simulink model "CHinf"  (R2020b)
settings: Solver=ode45  StartTime=0.0  StopTime=10  FixedStep=0.01  MaxStep=0.01  RelTol=1e-3  EnableMultiTasking=on
undefined symbols (not defined in the file): B, J, K1, Ke, Kt, Ra
settings Model: Creator=Harryth  LastModifiedBy=andre
settings DataIOCC: LimitDataPoints=on  SaveFormat=Array  SignalLoggingSaveFormat=ModelDataLogs  ReturnWorkspaceOutputs=off
settings OptimizationCC: ExpressionDepthLimit=2147483647  LifeSpan=inf
settings DebuggingCC: UnderspecifiedInitializationDetection=Classic  MergeDetectMultiDrivingBlocksExec=none  SolverPrmCheckMsg=warning  FcnCallInpInsideContextMsg=warning  StateNameClashWarn=warning  SFUnexpectedBacktrackingDiag=warning  SFNoUnconditionalDefaultTransitionDiag=warning  SFExecutionAtInitializationDiag=none  ArithmeticOperatorsInVariantConditions=warning
settings HardwareCC: ProdBitPerPointer=32  ProdBitPerSizeT=32  ProdBitPerPtrDiffT=32  ProdLargestAtomicFloat=None  ProdIntDivRoundTo=Undefined  ProdEndianess=Unspecified  ProdWordSize=32  ProdHWDeviceType=32-bit Generic
settings ModelReferenceCC: PropagateSignalLabelsOutOfModel=off
settings SFSimCC: SimUseLocalCustomCode=off  CustomCodeUndefinedFunction=UseInterfaceOnly
settings RTWCC: RTWUseLocalCustomCode=off
settings CodeAppCC: StateflowObjectComments=on
settings GRTTargetCC: TargetLangStandard=C89/C90 (ANSI)  CombineOutputUpdateFcns=off  GRTInterface=on
settings ConfigComp: CovMetricSettings=dw  CovSaveCumulativeToWorkspaceVar=on  CovSaveSingleToWorkspaceVar=on  CovExternalEMLEnable=off

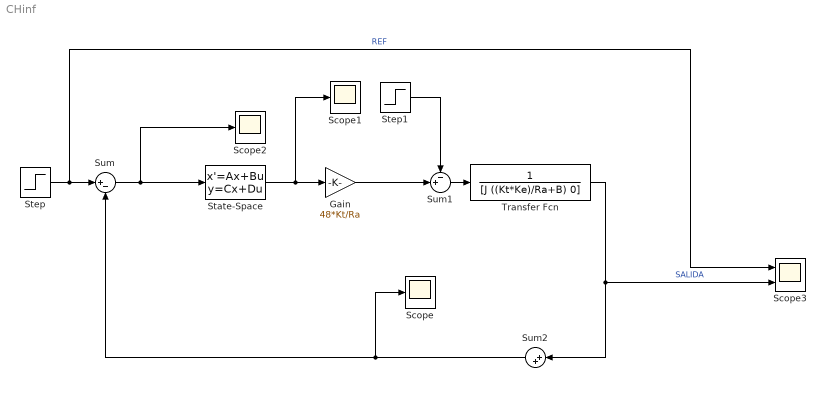
== system CHinf ==
  Gain : Gain  Gain=48*Kt/Ra
  Scope : Scope
  Scope1 : Scope
  Scope2 : Scope
  Scope3 : Scope  NumInputPorts=2
  State-Space : StateSpace  A=K1.a  B=K1.b  C=K1.c  D=K1.d  InitialCondition=0
  Step : Step  SampleTime=0
  Step1 : Step  Time=5  SampleTime=0
  Sum : Sum  Inputs=|+-
  Sum1 : Sum  Inputs=-+|
  Sum2 : Sum  Inputs=|++
  Transfer Fcn : TransferFcn  Numerator=1  Denominator=[J ((Kt*Ke)/Ra+B) 0]
  wires:
  Step/1 -> Scope3/1, Sum/1  "REF"
  Sum/1 -> Scope2/1, State-Space/1
  Gain/1 -> Sum1/2
  Sum1/1 -> Transfer Fcn/1
  Sum2/1 -> Sum/2, Scope/1
  Transfer Fcn/1 -> Sum2/1, Scope3/2  "SALIDA"
  Step1/1 -> Sum1/1
  State-Space/1 -> Gain/1, Scope1/1
